simulink model "SF106A_MotRplCoggCfg"  (R2013b)
settings: Solver=FixedStepDiscrete  SolverMode=SingleTasking  StartTime=0.0  StopTime=1  FixedStep=0.002  RelTol=1e-3
undefined symbols (not defined in the file): ARCHGLBPRM_2PI_ULS_F32, ARCHGLBPRM_FLOATZEROTHD_ULS_F32, ARCHGLBPRM_HALFSQRT3_ULS_F32, COGGORDER1_CNT_U16, COGGORDER2_CNT_U16, COGGORDER3_CNT_U16, magnitude, MotCtrlPrmEstimnMotBackEmfConNom, MotRplCoggCfgMotAgTiDly, MotRplCoggCfgMotCurrDaxRplBilnrSeln, MotRplCoggCfgMotCurrQaxRpl, MotRplCoggCfgMotTqRplOrder1X, MotRplCoggCfgMotTqRplOrder1Y, MotRplCoggCfgMotTqRplOrder2X, MotRplCoggCfgMotTqRplOrder2Y, MotRplCoggCfgMotTqRplOrder3X, MotRplCoggCfgMotTqRplOrder3Y, MotRplCoggCmdHrmncOrder1Elec, MotRplCoggCmdHrmncOrder2Elec, MotRplCoggCmdHrmncOrder3Elec, NvmGetErrSts1, ONEOVER2_ULS_F32, SysGlbPrmMotPoleCnt, THREEOVER8_ULS_F32
libraries: NxtrLim x20, FixdToFloat x12, FloatToFixd x6, BilnrIntrpnCmnX x6, BilnrIntrpnCmnXDyn x6, NxtrMath x6, NxtrAbslt x5, NxtrNvM x3, simulink x2, NxtrSign x2
(part 1 of 3)
settings Model: Creator=BZHF94  LastModifiedBy=BZHF94
settings SolverCC: AutoInsertRateTranBlk=on  InsertRTBMode=Always
settings DataIOCC: LimitDataPoints=off  SaveFormat=Structure  ReturnWorkspaceOutputs=on
settings OptimizationCC: BlockReduction=off  InlineParams=on  ZeroExternalMemoryAtStartup=off  ZeroInternalMemoryAtStartup=off  OptimizeModelRefInitCode=on  LifeSpan=1
settings DebuggingCC: SignalInfNanChecking=error  SignalRangeChecking=warning  UnderspecifiedInitializationDetection=Simplified  SolverPrmCheckMsg=error  InheritedTsInSrcMsg=error  DiscreteInheritContinuousMsg=error  SingleTaskRateTransMsg=error  TasksWithSamePriorityMsg=error  SigSpecEnsureSampleTimeMsg=error  CheckMatrixSingularityMsg=error  ParameterUnderflowMsg=error  ParameterPrecisionLossMsg=error  ParameterTunabilityLossMsg=error  FixptConstUnderflowMsg=warning  FixptConstOverflowMsg=warning  VectorMatrixConversionMsg=error  SignalLabelMismatchMsg=error  UnconnectedInputMsg=error  UnconnectedOutputMsg=error  UnconnectedLineMsg=error  SFcnCompatibilityMsg=error  UniqueDataStoreMsg=warning  BusObjectLabelMismatch=error  RootOutportRequireBusObject=error  AssertControl=DisableAll  ModelReferenceIOMsg=error  ModelReferenceVersionMismatchMessage=warning  ModelReferenceIOMismatchMessage=error  ModelReferenceCSMismatchMessage=warning  ModelReferenceDataLoggingMessage=error  StateNameClashWarn=warning  StrictBusMsg=ErrorOnBusTreatedAsVector  NonBusSignalsTreatedAsBus=error  SFUnexpectedBacktrackingDiag=error  SFInvalidInputDataAccessInChartInitDiag=error  SFNoUnconditionalDefaultTransitionDiag=error  SFTransitionOutsideNaturalParentDiag=error  SFUnconditionalTransitionShadowingDiag=error  SFUndirectedBroadcastEventsDiag=error
settings ModelReferenceCC: ModelReferenceNumInstancesAllowed=Single
settings RTWCC: SystemTargetFile=autosar.tlc  GenCodeOnly=on  TemplateMakefile=ert_default_tmf  Description=AUTOSAR  GenerateReport=on  ProcessScript=autosar_make_rtw_hook  LaunchReport=on
settings CodeAppCC: GenerateComments=off  IgnoreCustomStorageClasses=off  CustomSymbolStrType=$N$R$M  CustomSymbolStrBlkIO=$N$M  SimulinkBlockComments=off
settings STFCustomTargetCC: ParMdlRefBuildCompliant=on  CompOptLevelCompliant=on  IncludeMdlTerminateFcn=off  CombineOutputUpdateFcns=on  SuppressErrorStatus=on  ERTFirstTimeCompliant=on  ERTCustomFileBanners=on  SupportNonFinite=off  SupportComplex=off  SupportContinuousTime=off  SupportNonInlinedSFcns=off  MATLABClassNameForMDSCustomization=Simulink.SoftwareTarget.ERTCustomization  AutosarCompliant=on  GRTInterface=off  SystemTargetFile=autosar.tlc
settings ERTTargetCC: CodeReplacementLibrary=ANSI_C  ConcurrentExecutionCompliant=off  IncludeMdlTerminateFcn=off  SuppressErrorStatus=on  SupportNonFinite=off  SupportComplex=off  ModelStepFunctionPrototypeControlCompliant=off  CPPClassGenCompliant=off  AutosarCompliant=on  InlinedParameterPlacement=NonHierarchical  ERTCustomFileTemplate=example_file_process.tlc  EnableUserReplacementTypes=on

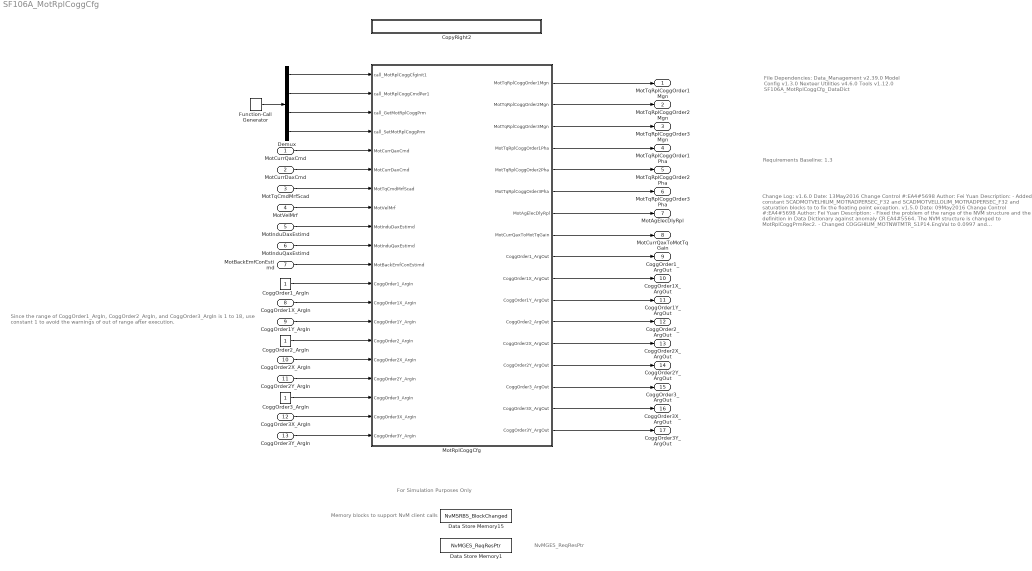
== system SF106A_MotRplCoggCfg ==
  note: Since the range of CoggOrder1_ArgIn, CoggOrder2_ArgIn, and CoggOrder3_ArgIn is 1 to 18,
      | use constant 1 to avoid the warnings of out of range after execution.
  note: NvMGES_ReqResPtr
  note: Change Log:
      |
      | v1.6.0
      | Date: 13May2016
      | Change Control #:EA4#5698
      | Author: Fei Yuan
      | Description:
      | - Added constant SCADMOTVELHILIM_MOTRADPERSEC_F32 and
      |   SCADMOTVELLOLIM_MOTRADPERSEC_F32 and saturation blocks to
      |   to fix the floating point exception.
      |
      | v1.5.0
      | Date: 09May2016
      | Change Control #:EA4#5698
      | Author: Fei Yuan
      | Description:
      | - Fixed the problem of the range of the NVM structure and the definition in Data
      |   Dictionary against anomaly CR EA4#5564. The NVM structure is changed to
      |   MotRplCoggPrmRec2.
      | - Changed COGGHILIM_MOTNWTMTR_S1P14.EngVal to 0.0997 and
      |   COGGLOLIM_MOTNWTMTR_S1P14.EngVal to -0.0997.
      |
      | v1.4.0
      | Date: 13April2016
      | Change Control #:EA4#5285
      | Author: Siva
      | Description:
      | - Updated GetErrorStatus library as per the new library block.
      |
      | v1.3.0
      | Date: 08April2016
      | Change Control #:EA4#4984
      | Author: Siva, Fei
      | Description:
      | - Updated initialization of q-axis current to torque multiplier.
      | - Added saturation blocks before signals writing to the NVM
      | - Changed the EngMin of the output signals MotTqRplCoggOrder1Mgn,
      |    MotTqRplCoggOrder2Mgn,and MotTqRplCoggOrder3Mgn to 0.
      |
      | v1.2.0
      | Date: 10February2016
      | Change Control #:EA4#2995
      | Author: Fei Yuan
      | Description:
      | - Fix the mistake two signals were connected improper
      |
      | v1.1.0
      | Date: 10February2016
      | Change Control #:EA4#2995
      | Author: Fei Yuan
      | Description:
      |  - Change MotRplCoggCfgMotCurrQaxRpl.EngVal to be 'Strictly_Increasing'.
      | - Add a condition when phase angles are over 2*PI to the wrapping blocks.
      | - Change MotRplCoggCfgMotVelBilnrSeln.EngDT to u16p0.
      | - Change SysGlbPrmMotPoleCnt.EngDT to u08.
      | - Add 'MotRplCoggCfgInit1' to SetRamBlockStatus.CallLocation.
      | - Minors changes for the sign block and saturation blocks for the phase angle.
      |
      | v1.0.0
      | Date: 01February2016
      | Change Control #: EA4#2995
      | Author: Fei Yuan
      | Description:
      |
      | - Initial release for EA4 based on version 1 in EA3.
  note: File Dependencies:
      |
      | Data_Management v2.39.0
      | Model Config v1.3.0
      | Nexteer Utilities v4.6.0
      | Tools v1.12.0
      |
      | SF106A_MotRplCoggCfg_DataDict
  note: Requirements Baseline: 1.3
  note: For Simulation Purposes Only
  note: Memory blocks to support NvM client calls
  MotCurrQaxCmd : Inport  RequirementInfo={} %GIDa_757f3847_d3ad_44cc_8eaf_0a9c1d691541
  MotCurrDaxCmd : Inport  RequirementInfo={} %GIDa_0b23bec1_bf45_466e_8236_41c598e6e599  Port=2
  MotTqCmdMrfScad : Inport  RequirementInfo={} %GIDa_35e7476b_4428_4fb9_921f_11cfc0c68159  Port=3
  MotVelMrf : Inport  RequirementInfo={} %GIDa_0381d354_c266_49b7_bf6e_c0e5b5782f60  Port=4
  MotInduDaxEstimd : Inport  RequirementInfo={} %GIDa_31de6d15_738a_4c67_a33c_60a1b9f25ce8  Port=5
  MotInduQaxEstimd : Inport  RequirementInfo={} %GIDa_f4a95a4b_a239_45ac_8ee5_2f92705b7f00  Port=6
  MotBackEmfConEstimd : Inport  RequirementInfo={} %GIDa_b2d97464_0b0a_4f6a_8955_43c989276f52  Port=7
  CoggOrder1X_ArgIn : Inport  Port=8
  CoggOrder1Y_ArgIn : Inport  Port=9
  CoggOrder2X_ArgIn : Inport  Port=10
  CoggOrder2Y_ArgIn : Inport  Port=11
  CoggOrder3X_ArgIn : Inport  Port=12
  CoggOrder3Y_ArgIn : Inport  Port=13
  CoggOrder1_ArgIn : Constant  OutDataTypeStr=uint16
  CoggOrder2_ArgIn : Constant  OutDataTypeStr=uint16
  CoggOrder3_ArgIn : Constant  OutDataTypeStr=uint16
  CopyRight2 : Subsystem  Description=|  mask(Copyright Information){none=on}
      | Copyright info block.                                               
      |                                                                     
      | Place copyright information at the top of every subsystem in design.
      mask prompts: none "No parameters"
      mask help: Place copyright information at the top of every subsystem in design.
      mask Display:
      | NxtrConf = 'Nexteer Confidential';
      | 
      | sys = bdroot; %handle for the current model ("system")
      | first = get_param(sys,'Created');
      | if(isempty(first))
      |     first = datestr(now,'yyyy');
      | else
      |     first = first(end-3:end);  %year is last four digits
      | end
      | 
      | last = get_param(sys,'LastModifiedDate');
      | if isempty(last)
      |     last = datestr(now,'yyyy');
      | else
      |     last = last(end-3:end);
      | end
      | 
      | if strcmp(first,last)
      |     fprintf('%s -- Copyright %s Nexteer',NxtrConf,first)
      | else
      |     fprintf('%s -- %s%s- %s Nexteer',NxtrConf,char(169),first,last)
      | end
  Data Store Memory1 : DataStoreMemory  DataStoreName=NvMGES_ReqResPtr  VectorParams1D=off
  Data Store Memory15 : DataStoreMemory  DataStoreName=NvMSRBS_BlockChanged  VectorParams1D=off
  Demux : Demux
  Function-Call Generator : simulink/Ports & Subsystems/Function-Call Generator  sample_time=1  numberOfIterations=1
  MotRplCoggCfg : Subsystem
  MotTqRplCoggOrder1Mgn : Outport  RequirementInfo={} %GIDa_0074686f_58d1_4901_a648_e28fd3eee3e7
  MotTqRplCoggOrder2Mgn : Outport  RequirementInfo={} %GIDa_99ad5412_b895_4313_9103_43633f08367a  Port=2
  MotTqRplCoggOrder3Mgn : Outport  RequirementInfo={} %GIDa_1162b2c3_d0bc_4efd_9968_0b9bdd62f2e0  Port=3
  MotTqRplCoggOrder1Pha : Outport  RequirementInfo={} %GIDa_e6635fbe_e43a_43a5_89b9_a832fe06509c  Port=4
  MotTqRplCoggOrder2Pha : Outport  RequirementInfo={} %GIDa_61383b7c_41e0_4245_ae1c_dbd664fb1655  Port=5
  MotTqRplCoggOrder3Pha : Outport  RequirementInfo={} %GIDa_2dd3ffc4_875a_4293_abc5_e3f7f6323b90  Port=6
  MotAgElecDlyRpl : Outport  RequirementInfo={} %GIDa_f8b0ade5_409e_4381_a98c_744f31aa9057  Port=7
  MotCurrQaxToMotTqGain : Outport  RequirementInfo={} %GIDa_da3becb4_ca59_41dc_ace4_45d9d90174a0  Port=8
  CoggOrder1_ArgOut : Outport  Port=9
  CoggOrder1X_ArgOut : Outport  Port=10
  CoggOrder1Y_ArgOut : Outport  Port=11
  CoggOrder2_ArgOut : Outport  Port=12
  CoggOrder2X_ArgOut : Outport  Port=13
  CoggOrder2Y_ArgOut : Outport  Port=14
  CoggOrder3_ArgOut : Outport  Port=15
  CoggOrder3X_ArgOut : Outport  Port=16
  CoggOrder3Y_ArgOut : Outport  Port=17
  wires:
  CoggOrder1_ArgIn/1 -> MotRplCoggCfg/12(CoggOrder1_ArgIn)
  CoggOrder2_ArgIn/1 -> MotRplCoggCfg/15(CoggOrder2_ArgIn)
  CoggOrder3_ArgIn/1 -> MotRplCoggCfg/18(CoggOrder3_ArgIn)
  MotRplCoggCfg/1(MotTqRplCoggOrder1Mgn) -> MotTqRplCoggOrder1Mgn/1
  MotRplCoggCfg/2(MotTqRplCoggOrder2Mgn) -> MotTqRplCoggOrder2Mgn/1
  MotRplCoggCfg/3(MotTqRplCoggOrder3Mgn) -> MotTqRplCoggOrder3Mgn/1
  MotRplCoggCfg/4(MotTqRplCoggOrder1Pha) -> MotTqRplCoggOrder1Pha/1
  MotRplCoggCfg/5(MotTqRplCoggOrder2Pha) -> MotTqRplCoggOrder2Pha/1
  MotRplCoggCfg/6(MotTqRplCoggOrder3Pha) -> MotTqRplCoggOrder3Pha/1
  MotRplCoggCfg/7(MotAgElecDlyRpl) -> MotAgElecDlyRpl/1
  MotRplCoggCfg/8(MotCurrQaxToMotTqGain) -> MotCurrQaxToMotTqGain/1
  MotRplCoggCfg/9(CoggOrder1_ArgOut) -> CoggOrder1_ArgOut/1
  MotRplCoggCfg/10(CoggOrder1X_ArgOut) -> CoggOrder1X_ArgOut/1
  MotRplCoggCfg/11(CoggOrder1Y_ArgOut) -> CoggOrder1Y_ArgOut/1
  MotRplCoggCfg/12(CoggOrder2_ArgOut) -> CoggOrder2_ArgOut/1
  MotRplCoggCfg/13(CoggOrder2X_ArgOut) -> CoggOrder2X_ArgOut/1
  MotRplCoggCfg/14(CoggOrder2Y_ArgOut) -> CoggOrder2Y_ArgOut/1
  MotRplCoggCfg/15(CoggOrder3_ArgOut) -> CoggOrder3_ArgOut/1
  MotRplCoggCfg/16(CoggOrder3X_ArgOut) -> CoggOrder3X_ArgOut/1
  MotRplCoggCfg/17(CoggOrder3Y_ArgOut) -> CoggOrder3Y_ArgOut/1
  MotCurrDaxCmd/1 -> MotRplCoggCfg/6(MotCurrDaxCmd)
  MotCurrQaxCmd/1 -> MotRplCoggCfg/5(MotCurrQaxCmd)
  MotTqCmdMrfScad/1 -> MotRplCoggCfg/7(MotTqCmdMrfScad)
  MotVelMrf/1 -> MotRplCoggCfg/8(MotVelMrf)
  MotInduDaxEstimd/1 -> MotRplCoggCfg/9(MotInduDaxEstimd)
  MotInduQaxEstimd/1 -> MotRplCoggCfg/10(MotInduQaxEstimd)
  MotBackEmfConEstimd/1 -> MotRplCoggCfg/11(MotBackEmfConEstimd)
  CoggOrder1X_ArgIn/1 -> MotRplCoggCfg/13(CoggOrder1X_ArgIn)
  CoggOrder1Y_ArgIn/1 -> MotRplCoggCfg/14(CoggOrder1Y_ArgIn)
  CoggOrder2X_ArgIn/1 -> MotRplCoggCfg/16(CoggOrder2X_ArgIn)
  CoggOrder2Y_ArgIn/1 -> MotRplCoggCfg/17(CoggOrder2Y_ArgIn)
  CoggOrder3X_ArgIn/1 -> MotRplCoggCfg/19(CoggOrder3X_ArgIn)
  CoggOrder3Y_ArgIn/1 -> MotRplCoggCfg/20(CoggOrder3Y_ArgIn)
  Demux/1 -> MotRplCoggCfg/1(call_MotRplCoggCfgInit1)
  Demux/2 -> MotRplCoggCfg/2(call_MotRplCoggCmdPer1)
  Function-Call Generator/1 -> Demux/1
  Demux/3 -> MotRplCoggCfg/3(call_GetMotRplCoggPrm)
  Demux/4 -> MotRplCoggCfg/4(call_SetMotRplCoggPrm)

== system SF106A_MotRplCoggCfg/CopyRight2 ==

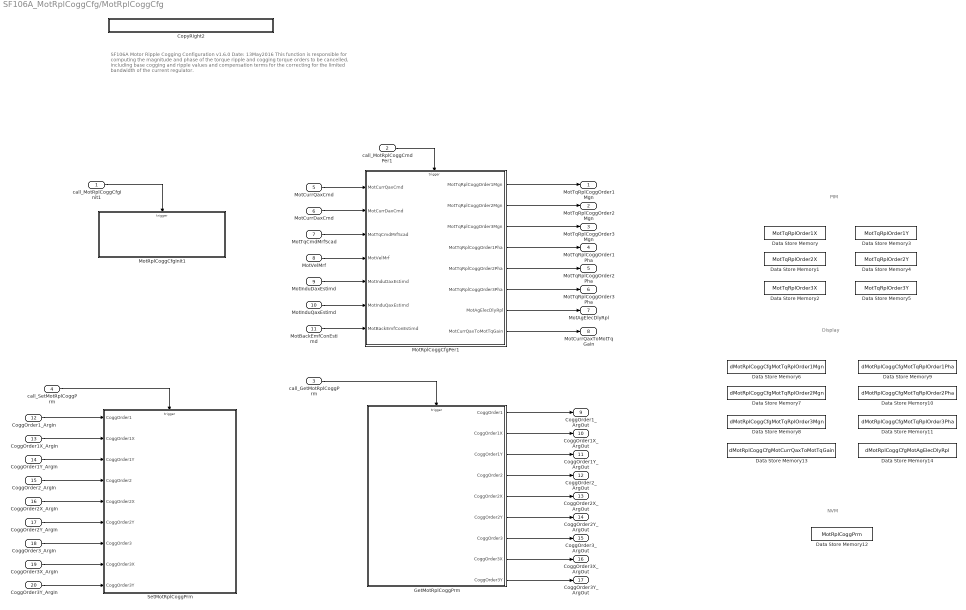
== system SF106A_MotRplCoggCfg/MotRplCoggCfg ==
  note: PIM
  note: SF106A  Motor Ripple Cogging Configuration
      | v1.6.0      Date: 13May2016
      |
      | This function is responsible for computing the magnitude and phase of the torque ripple and cogging torque
      | orders to be cancelled, including base cogging and ripple values and compensation terms for the correcting
      | for the limited bandwidth of the current regulator.
  note: Display
  note: NVM
  call_MotRplCoggCfgInit1 : Inport
  call_MotRplCoggCmdPer1 : Inport  RequirementInfo="{'linktype_rmi_doors' '0000bb45 (/E-STEER Core/SubSystem Specifications/Application Functions/SF99/SF106A Cogging and Ripple Configuration)' '#SF106A_52' 'true' 'REQ:  SF106A_52' '' } %GIDa_69adbc74_2cff_441d_948e_1d7a9b1e3618"  Port=2
  call_GetMotRplCoggPrm : Inport  Port=3
  call_SetMotRplCoggPrm : Inport  Port=4
  MotCurrQaxCmd : Inport  RequirementInfo="{'linktype_rmi_doors' '0000bb45 (/E-STEER Core/SubSystem Specifications/Application Functions/SF99/SF106A Cogging and Ripple Configuration)' '#SF106A_42' 'true' 'REQ:  SF106A_42' '' } %GIDa_5a05ee52_98b0_402f_8a8f_b325eaa6d628"  Port=5
  MotCurrDaxCmd : Inport  RequirementInfo="{'linktype_rmi_doors' '0000bb45 (/E-STEER Core/SubSystem Specifications/Application Functions/SF99/SF106A Cogging and Ripple Configuration)' '#SF106A_27' 'true' 'REQ:  SF106A_27' '' } %GIDa_163a6dc9_bd2b_42dd_b915_9d172b618666"  Port=6
  MotTqCmdMrfScad : Inport  RequirementInfo="{'linktype_rmi_doors' '0000bb45 (/E-STEER Core/SubSystem Specifications/Application Functions/SF99/SF106A Cogging and Ripple Configuration)' '#SF106A_45' 'true' 'REQ:  SF106A_45' '' } %GIDa_7dde8827_66c2_40f3_a684_d9cc8d489291"  Port=7
  MotVelMrf : Inport  RequirementInfo="{'linktype_rmi_doors' '0000bb45 (/E-STEER Core/SubSystem Specifications/Application Functions/SF99/SF106A Cogging and Ripple Configuration)' '#SF106A_44' 'true' 'REQ:  SF106A_44' '' } %GIDa_4dd0fc2d_0d8f_4817_a42b_2e08e466c057"  Port=8
  MotInduDaxEstimd : Inport  RequirementInfo="{'linktype_rmi_doors' '0000bb45 (/E-STEER Core/SubSystem Specifications/Application Functions/SF99/SF106A Cogging and Ripple Configuration)' '#SF106A_43' 'true' 'REQ:  SF106A_43' '' } %GIDa_7c7df466_71f9_4f77_bb21_b12736d8f067"  Port=9
  MotInduQaxEstimd : Inport  RequirementInfo="{'linktype_rmi_doors' '0000bb45 (/E-STEER Core/SubSystem Specifications/Application Functions/SF99/SF106A Cogging and Ripple Configuration)' '#SF106A_41' 'true' 'REQ:  SF106A_41' '' } %GIDa_a720e60c_03d7_4986_a5ea_3145b48a2e17"  Port=10
  MotBackEmfConEstimd : Inport  RequirementInfo="{'linktype_rmi_doors' '0000bb45 (/E-STEER Core/SubSystem Specifications/Application Functions/SF99/SF106A Cogging and Ripple Configuration)' '#SF106A_39' 'true' 'REQ:  SF106A_39' '' } %GIDa_8b974bc1_9d48_4040_bc20_b5d1a9e376c1"  Port=11
  CoggOrder1_ArgIn : Inport  Port=12
  CoggOrder1X_ArgIn : Inport  Port=13
  CoggOrder1Y_ArgIn : Inport  Port=14
  CoggOrder2_ArgIn : Inport  Port=15
  CoggOrder2X_ArgIn : Inport  Port=16
  CoggOrder2Y_ArgIn : Inport  Port=17
  CoggOrder3_ArgIn : Inport  Port=18
  CoggOrder3X_ArgIn : Inport  Port=19
  CoggOrder3Y_ArgIn : Inport  Port=20
  CopyRight2 : Subsystem  Description=|  mask(Copyright Information){none=on}
      | Copyright info block.                                               
      |                                                                     
      | Place copyright information at the top of every subsystem in design.
      mask prompts: none "No parameters"
      mask help: Place copyright information at the top of every subsystem in design.
      mask Display:
      | NxtrConf = 'Nexteer Confidential';
      | 
      | sys = bdroot; %handle for the current model ("system")
      | first = get_param(sys,'Created');
      | if(isempty(first))
      |     first = datestr(now,'yyyy');
      | else
      |     first = first(end-3:end);  %year is last four digits
      | end
      | 
      | last = get_param(sys,'LastModifiedDate');
      | if isempty(last)
      |     last = datestr(now,'yyyy');
      | else
      |     last = last(end-3:end);
      | end
      | 
      | if strcmp(first,last)
      |     fprintf('%s -- Copyright %s Nexteer',NxtrConf,first)
      | else
      |     fprintf('%s -- %s%s- %s Nexteer',NxtrConf,char(169),first,last)
      | end
  Data Store Memory : DataStoreMemory  DataStoreName=MotTqRplOrder1X  InitialValue=[]  VectorParams1D=off  StateMustResolveToSignalObject=on
  Data Store Memory1 : DataStoreMemory  DataStoreName=MotTqRplOrder2X  InitialValue=[]  VectorParams1D=off  StateMustResolveToSignalObject=on
  Data Store Memory10 : DataStoreMemory  DataStoreName=dMotRplCoggCfgMotTqRplOrder2Pha  StateMustResolveToSignalObject=on
  Data Store Memory11 : DataStoreMemory  DataStoreName=dMotRplCoggCfgMotTqRplOrder3Pha  StateMustResolveToSignalObject=on
  Data Store Memory12 : DataStoreMemory  DataStoreName=MotRplCoggPrm  InitialValue=[]  OutDataTypeStr=Bus: MotRplCoggPrmRec2  StateMustResolveToSignalObject=on
  Data Store Memory13 : DataStoreMemory  DataStoreName=dMotRplCoggCfgMotCurrQaxToMotTqGain  StateMustResolveToSignalObject=on
  Data Store Memory14 : DataStoreMemory  DataStoreName=dMotRplCoggCfgMotAgElecDlyRpl  StateMustResolveToSignalObject=on
  Data Store Memory2 : DataStoreMemory  DataStoreName=MotTqRplOrder3X  InitialValue=[]  VectorParams1D=off  StateMustResolveToSignalObject=on
  Data Store Memory3 : DataStoreMemory  DataStoreName=MotTqRplOrder1Y  InitialValue=[]  VectorParams1D=off  StateMustResolveToSignalObject=on
  Data Store Memory4 : DataStoreMemory  DataStoreName=MotTqRplOrder2Y  InitialValue=[]  VectorParams1D=off  StateMustResolveToSignalObject=on
  Data Store Memory5 : DataStoreMemory  DataStoreName=MotTqRplOrder3Y  InitialValue=[]  VectorParams1D=off  StateMustResolveToSignalObject=on
  Data Store Memory6 : DataStoreMemory  DataStoreName=dMotRplCoggCfgMotTqRplOrder1Mgn  StateMustResolveToSignalObject=on
  Data Store Memory7 : DataStoreMemory  DataStoreName=dMotRplCoggCfgMotTqRplOrder2Mgn  StateMustResolveToSignalObject=on
  Data Store Memory8 : DataStoreMemory  DataStoreName=dMotRplCoggCfgMotTqRplOrder3Mgn  StateMustResolveToSignalObject=on
  Data Store Memory9 : DataStoreMemory  DataStoreName=dMotRplCoggCfgMotTqRplOrder1Pha  StateMustResolveToSignalObject=on
  GetMotRplCoggPrm : Subsystem
  MotRplCoggCfgInit1 : Subsystem
  MotRplCoggCfgPer1 : Subsystem
  SetMotRplCoggPrm : Subsystem
  MotTqRplCoggOrder1Mgn : Outport  RequirementInfo="{'linktype_rmi_doors' '0000bb45 (/E-STEER Core/SubSystem Specifications/Application Functions/SF99/SF106A Cogging and Ripple Configuration)' '#SF106A_28' 'true' 'REQ:  SF106A_28' '' } %GIDa_79fab2f6_7c7b_44db_8523_44700579f2ce"
  MotTqRplCoggOrder2Mgn : Outport  RequirementInfo="{'linktype_rmi_doors' '0000bb45 (/E-STEER Core/SubSystem Specifications/Application Functions/SF99/SF106A Cogging and Ripple Configuration)' '#SF106A_47' 'true' 'REQ:  SF106A_47' '' } %GIDa_80d77d74_310d_460a_9930_56474fbf9f31"  Port=2
  MotTqRplCoggOrder3Mgn : Outport  RequirementInfo="{'linktype_rmi_doors' '0000bb45 (/E-STEER Core/SubSystem Specifications/Application Functions/SF99/SF106A Cogging and Ripple Configuration)' '#SF106A_50' 'true' 'REQ:  SF106A_50' '' } %GIDa_9e2c936d_c01a_490d_928f_f339b9cfb5aa"  Port=3
  MotTqRplCoggOrder1Pha : Outport  RequirementInfo="{'linktype_rmi_doors' '0000bb45 (/E-STEER Core/SubSystem Specifications/Application Functions/SF99/SF106A Cogging and Ripple Configuration)' '#SF106A_51' 'true' 'REQ:  SF106A_51' '' } %GIDa_17411a7b_2dd4_46aa_bb97_c41b28f019df"  Port=4
  MotTqRplCoggOrder2Pha : Outport  RequirementInfo="{'linktype_rmi_doors' '0000bb45 (/E-STEER Core/SubSystem Specifications/Application Functions/SF99/SF106A Cogging and Ripple Configuration)' '#SF106A_48' 'true' 'REQ:  SF106A_48' '' } %GIDa_0079c9a7_8844_4032_8bc3_ef4d9f3f9221"  Port=5
  MotTqRplCoggOrder3Pha : Outport  RequirementInfo="{'linktype_rmi_doors' '0000bb45 (/E-STEER Core/SubSystem Specifications/Application Functions/SF99/SF106A Cogging and Ripple Configuration)' '#SF106A_49' 'true' 'REQ:  SF106A_49' '' } %GIDa_79702522_322a_4356_96f6_c747a281e3ef"  Port=6
  MotAgElecDlyRpl : Outport  RequirementInfo="{'linktype_rmi_doors' '0000bb45 (/E-STEER Core/SubSystem Specifications/Application Functions/SF99/SF106A Cogging and Ripple Configuration)' '#SF106A_77' 'true' 'REQ:  SF106A_77' '' } %GIDa_91b44aef_782e_4909_91cc_efa6132885cc"  Port=7
  MotCurrQaxToMotTqGain : Outport  RequirementInfo="{'linktype_rmi_doors' '0000bb45 (/E-STEER Core/SubSystem Specifications/Application Functions/SF99/SF106A Cogging and Ripple Configuration)' '#SF106A_46' 'true' 'REQ:  SF106A_46' '' } %GIDa_1ae8a13f_399c_453a_9dee_6ff2a1b03975"  Port=8
  CoggOrder1_ArgOut : Outport  Port=9
  CoggOrder1X_ArgOut : Outport  Port=10
  CoggOrder1Y_ArgOut : Outport  Port=11
  CoggOrder2_ArgOut : Outport  Port=12
  CoggOrder2X_ArgOut : Outport  Port=13
  CoggOrder2Y_ArgOut : Outport  Port=14
  CoggOrder3_ArgOut : Outport  Port=15
  CoggOrder3X_ArgOut : Outport  Port=16
  CoggOrder3Y_ArgOut : Outport  Port=17
  wires:
  MotRplCoggCfgPer1/8(MotCurrQaxToMotTqGain) -> MotCurrQaxToMotTqGain/1
  call_MotRplCoggCfgInit1/1 -> MotRplCoggCfgInit1/Trigger
  call_MotRplCoggCmdPer1/1 -> MotRplCoggCfgPer1/Trigger
  MotRplCoggCfgPer1/1(MotTqRplCoggOrder1Mgn) -> MotTqRplCoggOrder1Mgn/1
  MotRplCoggCfgPer1/5(MotTqRplCoggOrder2Pha) -> MotTqRplCoggOrder2Pha/1
  MotTqCmdMrfScad/1 -> MotRplCoggCfgPer1/3(MotTqCmdMrfScad)
  MotInduDaxEstimd/1 -> MotRplCoggCfgPer1/5(MotInduDaxEstimd)
  MotVelMrf/1 -> MotRplCoggCfgPer1/4(MotVelMrf)
  MotCurrDaxCmd/1 -> MotRplCoggCfgPer1/2(MotCurrDaxCmd)
  MotRplCoggCfgPer1/6(MotTqRplCoggOrder3Pha) -> MotTqRplCoggOrder3Pha/1
  MotRplCoggCfgPer1/3(MotTqRplCoggOrder3Mgn) -> MotTqRplCoggOrder3Mgn/1
  MotRplCoggCfgPer1/2(MotTqRplCoggOrder2Mgn) -> MotTqRplCoggOrder2Mgn/1
  MotRplCoggCfgPer1/4(MotTqRplCoggOrder1Pha) -> MotTqRplCoggOrder1Pha/1
  MotCurrQaxCmd/1 -> MotRplCoggCfgPer1/1(MotCurrQaxCmd)
  MotInduQaxEstimd/1 -> MotRplCoggCfgPer1/6(MotInduQaxEstimd)
  call_GetMotRplCoggPrm/1 -> GetMotRplCoggPrm/Trigger
  call_SetMotRplCoggPrm/1 -> SetMotRplCoggPrm/Trigger
  GetMotRplCoggPrm/1(CoggOrder1) -> CoggOrder1_ArgOut/1
  GetMotRplCoggPrm/2(CoggOrder1X) -> CoggOrder1X_ArgOut/1
  GetMotRplCoggPrm/3(CoggOrder1Y) -> CoggOrder1Y_ArgOut/1
  GetMotRplCoggPrm/4(CoggOrder2) -> CoggOrder2_ArgOut/1
  GetMotRplCoggPrm/5(CoggOrder2X) -> CoggOrder2X_ArgOut/1
  GetMotRplCoggPrm/6(CoggOrder2Y) -> CoggOrder2Y_ArgOut/1
  GetMotRplCoggPrm/7(CoggOrder3) -> CoggOrder3_ArgOut/1
  GetMotRplCoggPrm/8(CoggOrder3X) -> CoggOrder3X_ArgOut/1
  GetMotRplCoggPrm/9(CoggOrder3Y) -> CoggOrder3Y_ArgOut/1
  MotRplCoggCfgPer1/7(MotAgElecDlyRpl) -> MotAgElecDlyRpl/1
  MotBackEmfConEstimd/1 -> MotRplCoggCfgPer1/7(MotBackEmfConEstimd)
  CoggOrder1_ArgIn/1 -> SetMotRplCoggPrm/1(CoggOrder1)
  CoggOrder1X_ArgIn/1 -> SetMotRplCoggPrm/2(CoggOrder1X)
  CoggOrder1Y_ArgIn/1 -> SetMotRplCoggPrm/3(CoggOrder1Y)
  CoggOrder2_ArgIn/1 -> SetMotRplCoggPrm/4(CoggOrder2)
  CoggOrder2X_ArgIn/1 -> SetMotRplCoggPrm/5(CoggOrder2X)
  CoggOrder2Y_ArgIn/1 -> SetMotRplCoggPrm/6(CoggOrder2Y)
  CoggOrder3_ArgIn/1 -> SetMotRplCoggPrm/7(CoggOrder3)
  CoggOrder3X_ArgIn/1 -> SetMotRplCoggPrm/8(CoggOrder3X)
  CoggOrder3Y_ArgIn/1 -> SetMotRplCoggPrm/9(CoggOrder3Y)

== system SF106A_MotRplCoggCfg/MotRplCoggCfg/CopyRight2 ==

== system SF106A_MotRplCoggCfg/MotRplCoggCfg/GetMotRplCoggPrm ==
  function : TriggerPort  TriggerType=function-call
  Data Store Read8 : DataStoreRead  RequirementInfo="{'linktype_rmi_doors' '0000bb45 (/E-STEER Core/SubSystem Specifications/Application Functions/SF99/SF106A Cogging and Ripple Configuration)' '#SF106A_33' 'true' 'REQ:  SF106A_33' '' } %GIDa_e2a562f6_d2aa_4ac1_94a6_2708492fb968"  DataStoreName=MotRplCoggPrm  DataStoreElements=MotRplCoggPrm.CoggOrder1#MotRplCoggPrm.CoggOrder1X#MotRplCoggPrm.CoggOrder1Y#MotRplCoggPrm.CoggOrder2#MotRplCoggPrm.CoggOrder2X#MotRplCoggPrm.CoggOrder2Y#MotRplCoggPrm.CoggOrder3#MotRplCoggPrm.CoggOrder3X#MotRplCoggPrm.CoggOrder3Y
  CoggOrder1 : Outport
  CoggOrder1X : Outport  Port=2
  CoggOrder1Y : Outport  Port=3
  CoggOrder2 : Outport  Port=4
  CoggOrder2X : Outport  Port=5
  CoggOrder2Y : Outport  Port=6
  CoggOrder3 : Outport  Port=7
  CoggOrder3X : Outport  Port=8
  CoggOrder3Y : Outport  Port=9
  wires:
  Data Store Read8/2 -> CoggOrder1X/1
  Data Store Read8/1 -> CoggOrder1/1
  Data Store Read8/9 -> CoggOrder3Y/1
  Data Store Read8/8 -> CoggOrder3X/1
  Data Store Read8/7 -> CoggOrder3/1
  Data Store Read8/4 -> CoggOrder2/1
  Data Store Read8/3 -> CoggOrder1Y/1
  Data Store Read8/5 -> CoggOrder2X/1
  Data Store Read8/6 -> CoggOrder2Y/1

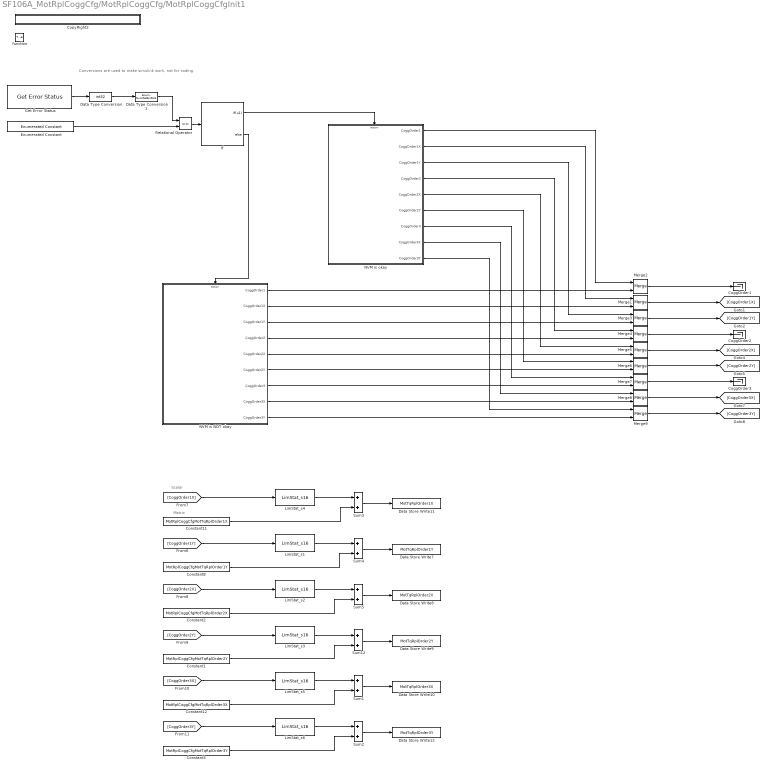
== system SF106A_MotRplCoggCfg/MotRplCoggCfg/MotRplCoggCfgInit1 ==
  note: Conversions are used to make simulink work, not for coding.
  note: Matrix
  note: Scalar
  function : TriggerPort  TriggerType=function-call
  CoggOrder1 : Terminator
  CoggOrder2 : Terminator
  CoggOrder3 : Terminator
  Constant1 : Constant  Value=MotRplCoggCfgMotTqRplOrder2Y
  Constant11 : Constant  Value=MotRplCoggCfgMotTqRplOrder1X
  Constant12 : Constant  Value=MotRplCoggCfgMotTqRplOrder3X
  Constant2 : Constant  Value=MotRplCoggCfgMotTqRplOrder2X
  Constant3 : Constant  Value=MotRplCoggCfgMotTqRplOrder3Y
  Constant8 : Constant  Value=MotRplCoggCfgMotTqRplOrder1Y
  CopyRight2 : Subsystem  Description=|  mask(Copyright Information){none=on}
      | Copyright info block.                                               
      |                                                                     
      | Place copyright information at the top of every subsystem in design.
      mask prompts: none "No parameters"
      mask help: Place copyright information at the top of every subsystem in design.
      mask Display:
      | NxtrConf = 'Nexteer Confidential';
      | 
      | sys = bdroot; %handle for the current model ("system")
      | first = get_param(sys,'Created');
      | if(isempty(first))
      |     first = datestr(now,'yyyy');
      | else
      |     first = first(end-3:end);  %year is last four digits
      | end
      | 
      | last = get_param(sys,'LastModifiedDate');
      | if isempty(last)
      |     last = datestr(now,'yyyy');
      | else
      |     last = last(end-3:end);
      | end
      | 
      | if strcmp(first,last)
      |     fprintf('%s -- Copyright %s Nexteer',NxtrConf,first)
      | else
      |     fprintf('%s -- %s%s- %s Nexteer',NxtrConf,char(169),first,last)
      | end
  Data Store Write10 : DataStoreWrite  DataStoreName=MotTqRplOrder3X
  Data Store Write11 : DataStoreWrite  DataStoreName=MotTqRplOrder1X
  Data Store Write12 : DataStoreWrite  DataStoreName=MotTqRplOrder3Y
  Data Store Write7 : DataStoreWrite  DataStoreName=MotTqRplOrder1Y
  Data Store Write8 : DataStoreWrite  DataStoreName=MotTqRplOrder2X
  Data Store Write9 : DataStoreWrite  DataStoreName=MotTqRplOrder2Y
  Data Type Conversion : DataTypeConversion  OutDataTypeStr=int32
  Data Type Conversion1 : DataTypeConversion  OutDataTypeStr=Enum: NvmGetErrSts1
  Enumerated Constant : simulink/Sources/Enumerated Constant  RequirementInfo="{'linktype_rmi_doors' '0000bb45 (/E-STEER Core/SubSystem Specifications/Application Functions/SF99/SF106A Cogging and Ripple Configuration)' '#SF106A_56' 'true' 'REQ:  SF106A_56' '' } %GIDa_049c6635_4162_44cf_9044_2549eb96868f"  OutDataTypeStr=Enum: NvmGetErrSts1  Value=NvmGetErrSts1.REQUEST_OK  SampleTime=inf
  Get Error Status : NxtrNvM/Get Error Status  RequirementInfo="{'linktype_rmi_doors' '0000bb45 (/E-STEER Core/SubSystem Specifications/Application Functions/SF99/SF106A Cogging and Ripple Configuration)' '#SF106A_56' 'true' 'REQ:  SF106A_56' '' } %GIDa_5785852d_b7e3_4bb7_b39f_00d1a50e86be"  FuncName=Get Error Status  NvMBlockName=MotRplCoggPrm  VoidFuncRtn=on  ReqResPtr_DSN=NvMGES_ReqResPtr  Return_DSN=NvMGES_Return
      settings: AttributesFormatString=%<FuncName>
  If : If  RequirementInfo="{'linktype_rmi_doors' '0000bb45 (/E-STEER Core/SubSystem Specifications/Application Functions/SF99/SF106A Cogging and Ripple Configuration)' '#SF106A_56' 'true' 'REQ:  SF106A_56' '' } %GIDa_e69cdbbe_6946_4c4a_a406_87bc5c36ef73"  IfExpression=u1
  LimStat_s{1..6} (6 alike) : NxtrLim/LimStat_s16  LoLim=COGGLOLIM_MOTNWTMTR_S1P14  HiLim=COGGHILIM_MOTNWTMTR_S1P14
      settings: AttributesFormatString=|
      | Low Limit: %<LoLim>
      | High Limit:%<HiLim>
  Merge{1..9} (9 alike) : Merge
  NVM is NOT okay : Subsystem  RequirementInfo="{'linktype_rmi_doors' '0000bb45 (/E-STEER Core/SubSystem Specifications/Application Functions/SF99/SF106A Cogging and Ripple Configuration)' '#SF106A_56' 'true' 'REQ:  SF106A_56' '' } %GIDa_89039b33_244c_4684_aea9_472cc9d16871"  TreatAsAtomicUnit=on
  NVM is okay : Subsystem  RequirementInfo="{'linktype_rmi_doors' '0000bb45 (/E-STEER Core/SubSystem Specifications/Application Functions/SF99/SF106A Cogging and Ripple Configuration)' '#SF106A_56' 'true' 'REQ:  SF106A_56' '' } %GIDa_57c12ef7_632e_42a8_a237_81adf7fb21f2"  TreatAsAtomicUnit=on
  Relational Operator : RelationalOperator  RequirementInfo="{'linktype_rmi_doors' '0000bb45 (/E-STEER Core/SubSystem Specifications/Application Functions/SF99/SF106A Cogging and Ripple Configuration)' '#SF106A_56' 'true' 'REQ:  SF106A_56' '' } %GIDa_53160261_4b9c_4422_9a16_4ee0d6230dc4"  Operator===  OutDataTypeStr=boolean
  Sum{1..5,12} (6 alike) : Sum
  wires:
  Get Error Status/1 -> Data Type Conversion/1
  If/1 -> NVM is okay/Action
  If/2 -> NVM is NOT okay/Action
  NVM is okay/1(CoggOrder1) -> Merge2/1
  NVM is NOT okay/1(CoggOrder1) -> Merge2/2
  NVM is okay/2(CoggOrder1X) -> Merge1/1
  NVM is NOT okay/2(CoggOrder1X) -> Merge1/2
  NVM is okay/3(CoggOrder1Y) -> Merge3/1
  NVM is NOT okay/3(CoggOrder1Y) -> Merge3/2
  NVM is okay/4(CoggOrder2) -> Merge4/1
  NVM is NOT okay/4(CoggOrder2) -> Merge4/2
  NVM is okay/5(CoggOrder2X) -> Merge5/1
  NVM is NOT okay/5(CoggOrder2X) -> Merge5/2
  NVM is okay/6(CoggOrder2Y) -> Merge6/1
  NVM is NOT okay/6(CoggOrder2Y) -> Merge6/2
  NVM is okay/7(CoggOrder3) -> Merge7/1
  NVM is NOT okay/7(CoggOrder3) -> Merge7/2
  NVM is NOT okay/8(CoggOrder3X) -> Merge8/2
  NVM is okay/8(CoggOrder3X) -> Merge8/1
  NVM is okay/9(CoggOrder3Y) -> Merge9/1
  NVM is NOT okay/9(CoggOrder3Y) -> Merge9/2
  Merge2/1 -> CoggOrder1/1
  Merge1/1 -> [CoggOrder1X]
  Merge3/1 -> [CoggOrder1Y]
  Merge4/1 -> CoggOrder2/1
  Merge5/1 -> [CoggOrder2X]
  Merge6/1 -> [CoggOrder2Y]
  Merge7/1 -> CoggOrder3/1
  Merge8/1 -> [CoggOrder3X]
  Merge9/1 -> [CoggOrder3Y]
  [CoggOrder1X] -> LimStat_s4/1
  [CoggOrder1Y] -> LimStat_s1/1
  LimStat_s4/1 -> Sum3/1
  Constant11/1 -> Sum3/2
  LimStat_s1/1 -> Sum4/1
  Constant8/1 -> Sum4/2
  [CoggOrder2X] -> LimStat_s2/1
  LimStat_s2/1 -> Sum5/1
  Constant2/1 -> Sum5/2
  LimStat_s3/1 -> Sum12/1
  Constant1/1 -> Sum12/2
  [CoggOrder3X] -> LimStat_s5/1
  LimStat_s5/1 -> Sum1/1
  Constant12/1 -> Sum1/2
  [CoggOrder3Y] -> LimStat_s6/1
  LimStat_s6/1 -> Sum2/1
  Constant3/1 -> Sum2/2
  Sum3/1 -> Data Store Write11/1
  Sum4/1 -> Data Store Write7/1
  Sum5/1 -> Data Store Write8/1
  Sum12/1 -> Data Store Write9/1
  Sum1/1 -> Data Store Write10/1
  Sum2/1 -> Data Store Write12/1
  [CoggOrder2Y] -> LimStat_s3/1
  Enumerated Constant/1 -> Relational Operator/2
  Relational Operator/1 -> If/1
  Data Type Conversion/1 -> Data Type Conversion1/1
  Data Type Conversion1/1 -> Relational Operator/1

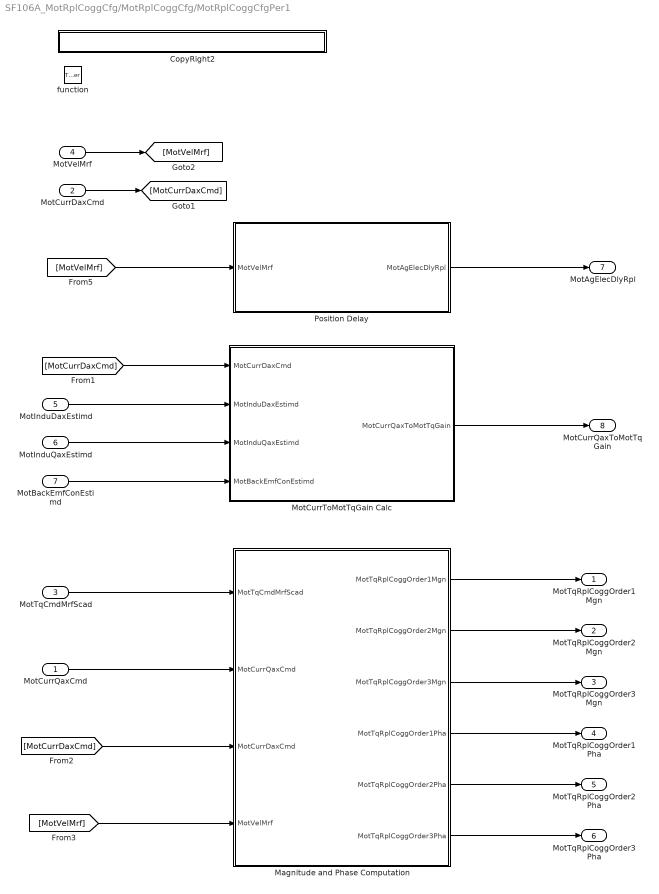
== system SF106A_MotRplCoggCfg/MotRplCoggCfg/MotRplCoggCfgPer1 ==
  MotCurrQaxCmd : Inport
  MotCurrDaxCmd : Inport  Port=2
  MotTqCmdMrfScad : Inport  Port=3
  MotVelMrf : Inport  Port=4
  MotInduDaxEstimd : Inport  Port=5
  MotInduQaxEstimd : Inport  Port=6
  MotBackEmfConEstimd : Inport  Port=7
  function : TriggerPort  TriggerType=function-call
  CopyRight2 : Subsystem  Description=|  mask(Copyright Information){none=on}
      | Copyright info block.                                               
      |                                                                     
      | Place copyright information at the top of every subsystem in design.
      mask prompts: none "No parameters"
      mask help: Place copyright information at the top of every subsystem in design.
      mask Display:
      | NxtrConf = 'Nexteer Confidential';
      | 
      | sys = bdroot; %handle for the current model ("system")
      | first = get_param(sys,'Created');
      | if(isempty(first))
      |     first = datestr(now,'yyyy');
      | else
      |     first = first(end-3:end);  %year is last four digits
      | end
      | 
      | last = get_param(sys,'LastModifiedDate');
      | if isempty(last)
      |     last = datestr(now,'yyyy');
      | else
      |     last = last(end-3:end);
      | end
      | 
      | if strcmp(first,last)
      |     fprintf('%s -- Copyright %s Nexteer',NxtrConf,first)
      | else
      |     fprintf('%s -- %s%s- %s Nexteer',NxtrConf,char(169),first,last)
      | end
  Magnitude and Phase Computation : Subsystem
  MotCurrToMotTqGain Calc : Subsystem
  Position Delay : Subsystem
  MotTqRplCoggOrder1Mgn : Outport
  MotTqRplCoggOrder2Mgn : Outport  Port=2
  MotTqRplCoggOrder3Mgn : Outport  Port=3
  MotTqRplCoggOrder1Pha : Outport  Port=4
  MotTqRplCoggOrder2Pha : Outport  Port=5
  MotTqRplCoggOrder3Pha : Outport  Port=6
  MotAgElecDlyRpl : Outport  Port=7
  MotCurrQaxToMotTqGain : Outport  Port=8
  wires:
  MotVelMrf/1 -> [MotVelMrf]
  MotInduDaxEstimd/1 -> MotCurrToMotTqGain Calc/2(MotInduDaxEstimd)
  MotInduQaxEstimd/1 -> MotCurrToMotTqGain Calc/3(MotInduQaxEstimd)
  MotBackEmfConEstimd/1 -> MotCurrToMotTqGain Calc/4(MotBackEmfConEstimd)
  MotCurrToMotTqGain Calc/1(MotCurrQaxToMotTqGain) -> MotCurrQaxToMotTqGain/1
  Position Delay/1(MotAgElecDlyRpl) -> MotAgElecDlyRpl/1
  [MotVelMrf] -> Position Delay/1(MotVelMrf)
  [MotCurrDaxCmd] -> MotCurrToMotTqGain Calc/1(MotCurrDaxCmd)
  MotCurrDaxCmd/1 -> [MotCurrDaxCmd]
  MotTqCmdMrfScad/1 -> Magnitude and Phase Computation/1(MotTqCmdMrfScad)
  MotCurrQaxCmd/1 -> Magnitude and Phase Computation/2(MotCurrQaxCmd)
  Magnitude and Phase Computation/1(MotTqRplCoggOrder1Mgn) -> MotTqRplCoggOrder1Mgn/1
  Magnitude and Phase Computation/2(MotTqRplCoggOrder2Mgn) -> MotTqRplCoggOrder2Mgn/1
  Magnitude and Phase Computation/3(MotTqRplCoggOrder3Mgn) -> MotTqRplCoggOrder3Mgn/1
  Magnitude and Phase Computation/4(MotTqRplCoggOrder1Pha) -> MotTqRplCoggOrder1Pha/1
  Magnitude and Phase Computation/5(MotTqRplCoggOrder2Pha) -> MotTqRplCoggOrder2Pha/1
  Magnitude and Phase Computation/6(MotTqRplCoggOrder3Pha) -> MotTqRplCoggOrder3Pha/1
  [MotCurrDaxCmd] -> Magnitude and Phase Computation/3(MotCurrDaxCmd)
  [MotVelMrf] -> Magnitude and Phase Computation/4(MotVelMrf)

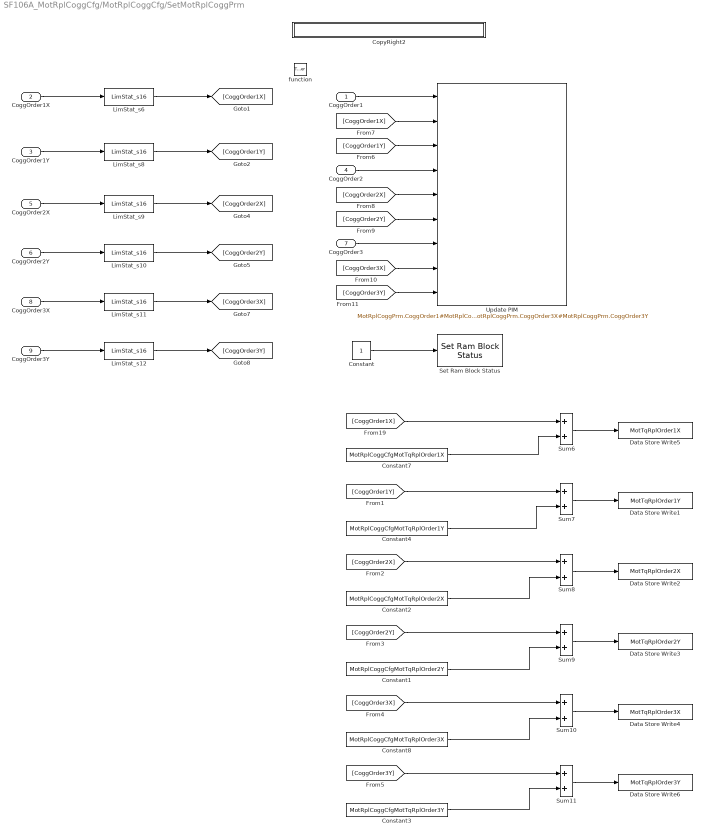
== system SF106A_MotRplCoggCfg/MotRplCoggCfg/SetMotRplCoggPrm ==
  CoggOrder1 : Inport
  CoggOrder1X : Inport  Port=2
  CoggOrder1Y : Inport  Port=3
  CoggOrder2 : Inport  Port=4
  CoggOrder2X : Inport  Port=5
  CoggOrder2Y : Inport  Port=6
  CoggOrder3 : Inport  Port=7
  CoggOrder3X : Inport  Port=8
  CoggOrder3Y : Inport  Port=9
  function : TriggerPort  TriggerType=function-call
  Constant : Constant  RequirementInfo="{'linktype_rmi_doors' '0000bb45 (/E-STEER Core/SubSystem Specifications/Application Functions/SF99/SF106A Cogging and Ripple Configuration)' '#SF106A_32' 'true' 'REQ:  SF106A_32' '' } %GIDa_5ec7b413_3022_404f_b73a_090841214aa3"  OutDataTypeStr=double
  Constant1 : Constant  Value=MotRplCoggCfgMotTqRplOrder2Y
  Constant2 : Constant  Value=MotRplCoggCfgMotTqRplOrder2X
  Constant3 : Constant  Value=MotRplCoggCfgMotTqRplOrder3Y
  Constant4 : Constant  Value=MotRplCoggCfgMotTqRplOrder1Y
  Constant7 : Constant  Value=MotRplCoggCfgMotTqRplOrder1X
  Constant8 : Constant  Value=MotRplCoggCfgMotTqRplOrder3X
  CopyRight2 : Subsystem  Description=|  mask(Copyright Information){none=on}
      | Copyright info block.                                               
      |                                                                     
      | Place copyright information at the top of every subsystem in design.
      mask prompts: none "No parameters"
      mask help: Place copyright information at the top of every subsystem in design.
      mask Display:
      | NxtrConf = 'Nexteer Confidential';
      | 
      | sys = bdroot; %handle for the current model ("system")
      | first = get_param(sys,'Created');
      | if(isempty(first))
      |     first = datestr(now,'yyyy');
      | else
      |     first = first(end-3:end);  %year is last four digits
      | end
      | 
      | last = get_param(sys,'LastModifiedDate');
      | if isempty(last)
      |     last = datestr(now,'yyyy');
      | else
      |     last = last(end-3:end);
      | end
      | 
      | if strcmp(first,last)
      |     fprintf('%s -- Copyright %s Nexteer',NxtrConf,first)
      | else
      |     fprintf('%s -- %s%s- %s Nexteer',NxtrConf,char(169),first,last)
      | end
  Data Store Write1 : DataStoreWrite  DataStoreName=MotTqRplOrder1Y
  Data Store Write2 : DataStoreWrite  DataStoreName=MotTqRplOrder2X
  Data Store Write3 : DataStoreWrite  DataStoreName=MotTqRplOrder2Y
  Data Store Write4 : DataStoreWrite  DataStoreName=MotTqRplOrder3X
  Data Store Write5 : DataStoreWrite  DataStoreName=MotTqRplOrder1X
  Data Store Write6 : DataStoreWrite  DataStoreName=MotTqRplOrder3Y
  LimStat_s{6,8..12} (6 alike) : NxtrLim/LimStat_s16  LoLim=COGGLOLIM_MOTNWTMTR_S1P14  HiLim=COGGHILIM_MOTNWTMTR_S1P14
      settings: AttributesFormatString=|
      | Low Limit: %<LoLim>
      | High Limit:%<HiLim>
  Set Ram Block Status : NxtrNvM/Set Ram Block Status  RequirementInfo="{'linktype_rmi_doors' '0000bb45 (/E-STEER Core/SubSystem Specifications/Application Functions/SF99/SF106A Cogging and Ripple Configuration)' '#SF106A_32' 'true' 'REQ:  SF106A_32' '' } %GIDa_c66198c4_a381_40cd_bb7f_8001ef97393a"  FuncName=Set Ram Block Status  NvMBlockName=MotRplCoggPrm  VoidFuncRtn=on  BlockChanged_DSN=NvMSRBS_BlockChanged  Return_DSN=NvMSRBS_Return
      settings: AttributesFormatString=%<FuncName>
  Sum{6..11} (6 alike) : Sum
  Update PIM : DataStoreWrite  RequirementInfo="{'linktype_rmi_doors' '0000bb45 (/E-STEER Core/SubSystem Specifications/Application Functions/SF99/SF106A Cogging and Ripple Configuration)' '#SF106A_32' 'true' 'REQ:  SF106A_32' '' } %GIDa_c247fc61_4ce4_4da4_ba94_7fa744912d87"  DataStoreName=MotRplCoggPrm  DataStoreElements=MotRplCoggPrm.CoggOrder1#MotRplCoggPrm.CoggOrder1X#MotRplCoggPrm.CoggOrder1Y#MotRplCoggPrm.CoggOrder2#MotRplCoggPrm.CoggOrder2X#MotRplCoggPrm.CoggOrder2Y#MotRplCoggPrm.CoggOrder3#MotRplCoggPrm.CoggOrder3X#MotRplCoggPrm.CoggOrder3Y
  wires:
  CoggOrder3X/1 -> LimStat_s11/1
  CoggOrder1Y/1 -> LimStat_s8/1
  CoggOrder2X/1 -> LimStat_s9/1
  CoggOrder3Y/1 -> LimStat_s12/1
  CoggOrder3/1 -> Update PIM/7
  CoggOrder2/1 -> Update PIM/4
  CoggOrder2Y/1 -> LimStat_s10/1
  Sum11/1 -> Data Store Write6/1
  Sum10/1 -> Data Store Write4/1
  Sum9/1 -> Data Store Write3/1
  Sum8/1 -> Data Store Write2/1
  Sum7/1 -> Data Store Write1/1
  Sum6/1 -> Data Store Write5/1
  Constant3/1 -> Sum11/2
  [CoggOrder3Y] -> Sum11/1
  Constant8/1 -> Sum10/2
  [CoggOrder3X] -> Sum10/1
  Constant1/1 -> Sum9/2
  [CoggOrder2Y] -> Sum9/1
  Constant2/1 -> Sum8/2
  [CoggOrder2X] -> Sum8/1
  Constant4/1 -> Sum7/2
  [CoggOrder1Y] -> Sum7/1
  Constant7/1 -> Sum6/2
  [CoggOrder1X] -> Sum6/1
  Constant/1 -> Set Ram Block Status/1
  CoggOrder1/1 -> Update PIM/1
  CoggOrder1X/1 -> LimStat_s6/1
  LimStat_s6/1 -> [CoggOrder1X]
  LimStat_s8/1 -> [CoggOrder1Y]
  LimStat_s9/1 -> [CoggOrder2X]
  LimStat_s10/1 -> [CoggOrder2Y]
  LimStat_s11/1 -> [CoggOrder3X]
  LimStat_s12/1 -> [CoggOrder3Y]
  [CoggOrder1X] -> Update PIM/2
  [CoggOrder1Y] -> Update PIM/3
  [CoggOrder2X] -> Update PIM/5
  [CoggOrder2Y] -> Update PIM/6
  [CoggOrder3X] -> Update PIM/8
  [CoggOrder3Y] -> Update PIM/9

== system SF106A_MotRplCoggCfg/MotRplCoggCfg/MotRplCoggCfgInit1/CopyRight2 ==

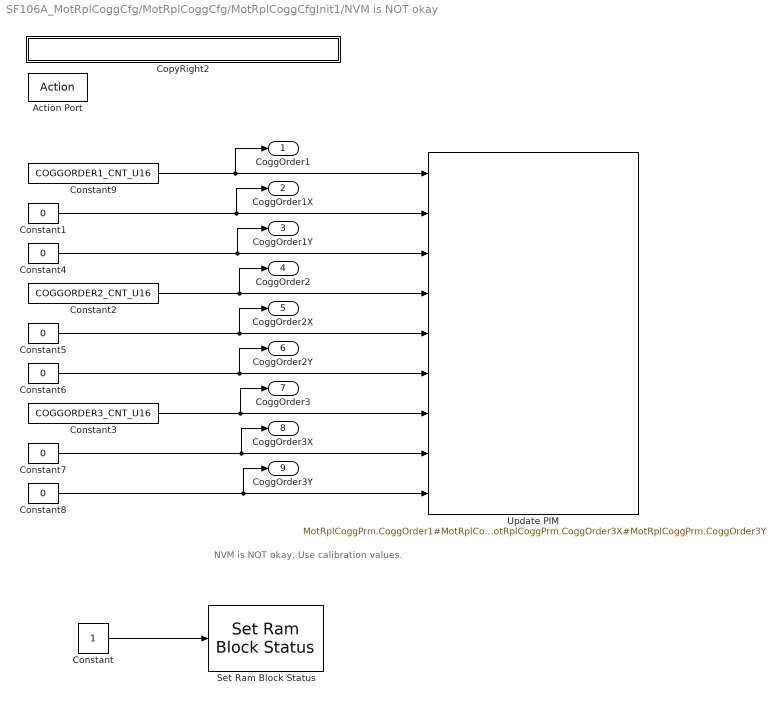
== system SF106A_MotRplCoggCfg/MotRplCoggCfg/MotRplCoggCfgInit1/NVM is NOT okay ==
  note: NVM is NOT okay. Use calibration values.
  Action Port : ActionPort  ActionType=else
  Constant : Constant  RequirementInfo="{'linktype_rmi_doors' '0000bb45 (/E-STEER Core/SubSystem Specifications/Application Functions/SF99/SF106A Cogging and Ripple Configuration)' '#SF106A_32' 'true' 'REQ:  SF106A_32' '' } %GIDa_88badfbe_a282_406c_a95c_f04d8f23c907"
  Constant1 : Constant  RequirementInfo={} %GIDa_8db4915b_ee3c_43ce_a6de_c08a14e2d8d9  Value=0  OutDataTypeStr=int16
      settings: AttributesFormatString=%<OutDataTypeStr>
  Constant2 : Constant  RequirementInfo={} %GIDa_45946a62_00db_48e4_a364_5f1880b825e2  Value=COGGORDER2_CNT_U16
  Constant3 : Constant  RequirementInfo={} %GIDa_97e171c7_9819_424e_ac7e_0acef4f870f8  Value=COGGORDER3_CNT_U16
  Constant4 : Constant  RequirementInfo={} %GIDa_8ae6259d_a884_4a89_96dc_6b58d99c59da  Value=0  OutDataTypeStr=int16
      settings: AttributesFormatString=%<OutDataTypeStr>
  Constant5 : Constant  RequirementInfo={} %GIDa_ae8168af_3c58_49c7_8b42_18041611ec17  Value=0  OutDataTypeStr=int16
      settings: AttributesFormatString=%<OutDataTypeStr>
  Constant6 : Constant  RequirementInfo={} %GIDa_2c4e09c0_949c_4ef2_9c8f_e2c962e14c31  Value=0  OutDataTypeStr=int16
      settings: AttributesFormatString=%<OutDataTypeStr>
  Constant7 : Constant  RequirementInfo={} %GIDa_cd0a1269_cd2b_4917_8273_55aafa709e41  Value=0  OutDataTypeStr=int16
      settings: AttributesFormatString=%<OutDataTypeStr>
  Constant8 : Constant  RequirementInfo={} %GIDa_8b948064_017d_418d_a632_66eec6e6c611  Value=0  OutDataTypeStr=int16
      settings: AttributesFormatString=%<OutDataTypeStr>
  Constant9 : Constant  RequirementInfo={} %GIDa_eabef9f5_252a_43d8_b1b1_e8370bbcbf50  Value=COGGORDER1_CNT_U16
  CopyRight2 : Subsystem  Description=|  mask(Copyright Information){none=on}
      | Copyright info block.                                               
      |                                                                     
      | Place copyright information at the top of every subsystem in design.
      mask prompts: none "No parameters"
      mask help: Place copyright information at the top of every subsystem in design.
      mask Display:
      | NxtrConf = 'Nexteer Confidential';
      | 
      | sys = bdroot; %handle for the current model ("system")
      | first = get_param(sys,'Created');
      | if(isempty(first))
      |     first = datestr(now,'yyyy');
      | else
      |     first = first(end-3:end);  %year is last four digits
      | end
      | 
      | last = get_param(sys,'LastModifiedDate');
      | if isempty(last)
      |     last = datestr(now,'yyyy');
      | else
      |     last = last(end-3:end);
      | end
      | 
      | if strcmp(first,last)
      |     fprintf('%s -- Copyright %s Nexteer',NxtrConf,first)
      | else
      |     fprintf('%s -- %s%s- %s Nexteer',NxtrConf,char(169),first,last)
      | end
  Set Ram Block Status : NxtrNvM/Set Ram Block Status  RequirementInfo="{'linktype_rmi_doors' '0000bb45 (/E-STEER Core/SubSystem Specifications/Application Functions/SF99/SF106A Cogging and Ripple Configuration)' '#SF106A_32' 'true' 'REQ:  SF106A_32' '' } %GIDa_66659699_c693_48e6_8b79_9140f0e4f0ee"  FuncName=Set Ram Block Status  NvMBlockName=MotRplCoggPrm  VoidFuncRtn=on  BlockChanged_DSN=NvMSRBS_BlockChanged  Return_DSN=NvMSRBS_Return
      settings: AttributesFormatString=%<FuncName>
  Update PIM : DataStoreWrite  RequirementInfo="{'linktype_rmi_doors' '0000bb45 (/E-STEER Core/SubSystem Specifications/Application Functions/SF99/SF106A Cogging and Ripple Configuration)' '#SF106A_32' 'true' 'REQ:  SF106A_32' '' } %GIDa_40d67f4b_8a98_4ada_ac75_a0740d8615d4"  DataStoreName=MotRplCoggPrm  DataStoreElements=MotRplCoggPrm.CoggOrder1#MotRplCoggPrm.CoggOrder1X#MotRplCoggPrm.CoggOrder1Y#MotRplCoggPrm.CoggOrder2#MotRplCoggPrm.CoggOrder2X#MotRplCoggPrm.CoggOrder2Y#MotRplCoggPrm.CoggOrder3#MotRplCoggPrm.CoggOrder3X#MotRplCoggPrm.CoggOrder3Y
  CoggOrder1 : Outport
  CoggOrder1X : Outport  Port=2
  CoggOrder1Y : Outport  Port=3
  CoggOrder2 : Outport  Port=4
  CoggOrder2X : Outport  Port=5
  CoggOrder2Y : Outport  Port=6
  CoggOrder3 : Outport  Port=7
  CoggOrder3X : Outport  Port=8
  CoggOrder3Y : Outport  Port=9
  wires:
  Constant/1 -> Set Ram Block Status/1
  Constant1/1 -> CoggOrder1X/1, Update PIM/2
  Constant4/1 -> CoggOrder1Y/1, Update PIM/3
  Constant5/1 -> CoggOrder2X/1, Update PIM/5
  Constant8/1 -> CoggOrder3Y/1, Update PIM/9
  Constant7/1 -> CoggOrder3X/1, Update PIM/8
  Constant6/1 -> CoggOrder2Y/1, Update PIM/6
  Constant9/1 -> CoggOrder1/1, Update PIM/1
  Constant2/1 -> CoggOrder2/1, Update PIM/4
  Constant3/1 -> CoggOrder3/1, Update PIM/7

== system SF106A_MotRplCoggCfg/MotRplCoggCfg/MotRplCoggCfgInit1/NVM is okay ==
  note: NVM is okay. Use stored value
  Action Port : ActionPort  ActionType=then
  CopyRight2 : Subsystem  Description=|  mask(Copyright Information){none=on}
      | Copyright info block.                                               
      |                                                                     
      | Place copyright information at the top of every subsystem in design.
      mask prompts: none "No parameters"
      mask help: Place copyright information at the top of every subsystem in design.
      mask Display:
      | NxtrConf = 'Nexteer Confidential';
      | 
      | sys = bdroot; %handle for the current model ("system")
      | first = get_param(sys,'Created');
      | if(isempty(first))
      |     first = datestr(now,'yyyy');
      | else
      |     first = first(end-3:end);  %year is last four digits
      | end
      | 
      | last = get_param(sys,'LastModifiedDate');
      | if isempty(last)
      |     last = datestr(now,'yyyy');
      | else
      |     last = last(end-3:end);
      | end
      | 
      | if strcmp(first,last)
      |     fprintf('%s -- Copyright %s Nexteer',NxtrConf,first)
      | else
      |     fprintf('%s -- %s%s- %s Nexteer',NxtrConf,char(169),first,last)
      | end
  Data Store Read2 : DataStoreRead  RequirementInfo="{'linktype_rmi_doors' '0000bb45 (/E-STEER Core/SubSystem Specifications/Application Functions/SF99/SF106A Cogging and Ripple Configuration)' '#SF106A_33' 'true' 'REQ:  SF106A_33' '' } %GIDa_bbb4bf81_36d2_4b89_8435_bb1b23410ef8"  DataStoreName=MotRplCoggPrm  DataStoreElements=MotRplCoggPrm.CoggOrder1#MotRplCoggPrm.CoggOrder1X#MotRplCoggPrm.CoggOrder1Y#MotRplCoggPrm.CoggOrder2#MotRplCoggPrm.CoggOrder2X#MotRplCoggPrm.CoggOrder2Y#MotRplCoggPrm.CoggOrder3#MotRplCoggPrm.CoggOrder3X#MotRplCoggPrm.CoggOrder3Y
  CoggOrder1 : Outport
  CoggOrder1X : Outport  Port=2
  CoggOrder1Y : Outport  Port=3
  CoggOrder2 : Outport  Port=4
  CoggOrder2X : Outport  Port=5
  CoggOrder2Y : Outport  Port=6
  CoggOrder3 : Outport  Port=7
  CoggOrder3X : Outport  Port=8
  CoggOrder3Y : Outport  Port=9
  wires:
  Data Store Read2/2 -> CoggOrder1X/1
  Data Store Read2/1 -> CoggOrder1/1
  Data Store Read2/9 -> CoggOrder3Y/1
  Data Store Read2/8 -> CoggOrder3X/1
  Data Store Read2/7 -> CoggOrder3/1
  Data Store Read2/4 -> CoggOrder2/1
  Data Store Read2/3 -> CoggOrder1Y/1
  Data Store Read2/5 -> CoggOrder2X/1
  Data Store Read2/6 -> CoggOrder2Y/1

== system SF106A_MotRplCoggCfg/MotRplCoggCfg/MotRplCoggCfgPer1/CopyRight2 ==
